simulink model "tremolo"  (R2025b)
settings: Solver=FixedStepDiscrete  StartTime=0.0  StopTime=inf  FixedStep=128/48000  RelTol=1e-3
model workspace (MATLAB code in the model file):
  | Gain_rt = Simulink.Parameter(1.0);
  | Bypass_rt = Simulink.Parameter(false);
undefined symbols (not defined in the file): Depth_rt
settings Model: Creator=linogarciamorales  LastModifiedBy=linogarciamorales
settings OptimizationCC: EnhancedBackFolding=on  PassReuseOutputArgsAs=Individual arguments  ZeroExternalMemoryAtStartup=off  ZeroInternalMemoryAtStartup=off  OptimizeBlockOrder=speed  DifferentSizesBufferReuse=on  OptimizationCustomize=off  EfficientTunableParamExpr=on
settings DebuggingCC: ParameterTunabilityLossMsg=error
settings SFSimCC: MATLABDynamicMemAlloc=off
settings RTWCC: SystemTargetFile=ert.tlc  GenCodeOnly=on  TemplateMakefile=ert_default_tmf  Description=Embedded Coder
settings CodeAppCC: ForceParamTrailComments=on  IgnoreCustomStorageClasses=off  OperatorAnnotations=on  SimulinkDataObjDesc=on  SFDataObjDesc=on  InsertBlockDesc=on
settings ERTTargetCC: InlinedParameterPlacement=Hierarchical  ERTCustomFileTemplate=example_file_process.tlc  TargetLangStandard=C99 (ISO)  GenerateSampleERTMain=on  SupportNonInlinedSFcns=on

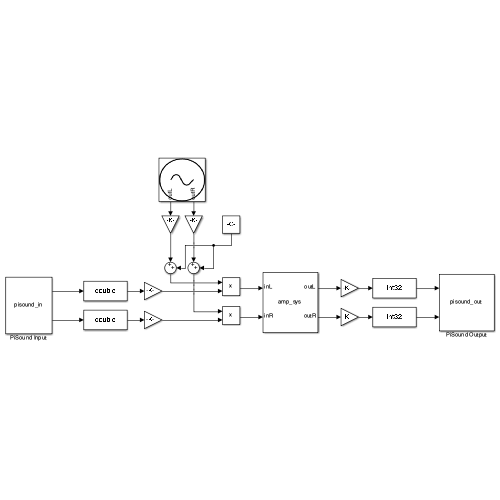
[thumbnail: Simulink's stored preview of the top-level diagram]
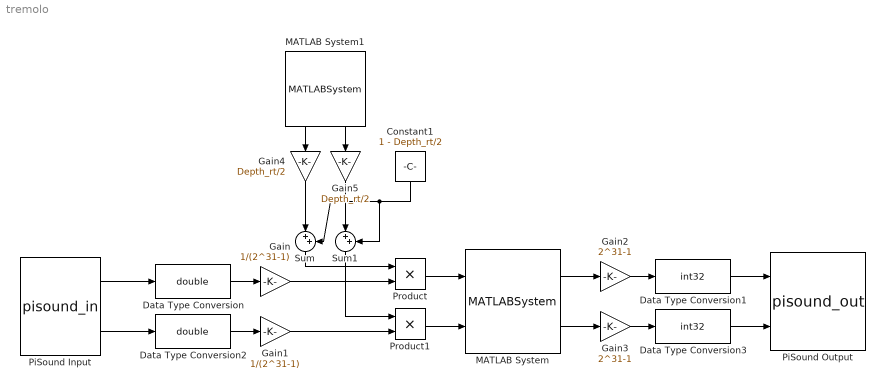
== system tremolo ==
  Constant1 : Constant  Value=1 - Depth_rt/2  OutDataTypeStr=double
  Data Type Conversion : DataTypeConversion  OutDataTypeStr=double  SaturateOnIntegerOverflow=off  RndMeth=Floor
  Data Type Conversion1 : DataTypeConversion  OutDataTypeStr=int32  SaturateOnIntegerOverflow=off  RndMeth=Floor
  Data Type Conversion2 : DataTypeConversion  OutDataTypeStr=double  SaturateOnIntegerOverflow=off  RndMeth=Floor
  Data Type Conversion3 : DataTypeConversion  OutDataTypeStr=int32  SaturateOnIntegerOverflow=off  RndMeth=Floor
  Gain : Gain  Gain=1/(2^31-1)
  Gain1 : Gain  Gain=1/(2^31-1)
  Gain2 : Gain  Gain=2^31-1
  Gain3 : Gain  Gain=2^31-1
  Gain4 : Gain  Gain=Depth_rt/2  ParamDataTypeStr=double
  Gain5 : Gain  Gain=Depth_rt/2  ParamDataTypeStr=double
  MATLAB System : MATLABSystem  System=amp_sys  Fs=48000  Gain=Gain_rt  Bypass=Bypass_rt  SimulateUsing=Code generation
      mask Type: amp_sys
  MATLAB System1 : MATLABSystem  System=osc_sys  N=128  Fs=48000  OutMaxL=4096  InFixL=1024  A=1  F=Rate_rt  iPhase=iPhase_rt  WaveSel=WaveSel_rt  SimulateUsing=Code generation
      mask Type: osc_sys
  PiSound Input : S-Function  FunctionName=pisound_in  Parameters=48000, 128, 0  SFunctionDeploymentMode=off  EnableBusSupport=off
  PiSound Output : S-Function  FunctionName=pisound_out  Parameters=48000, 128, 0  SFunctionDeploymentMode=off  EnableBusSupport=off
  Product : Product  OutDataTypeStr=double
  Product1 : Product  OutDataTypeStr=double
  Sum : Sum  Inputs=|++  OutDataTypeStr=double
  Sum1 : Sum  Inputs=|++  OutDataTypeStr=double
  wires:
  PiSound Input/1 -> Data Type Conversion/1
  Data Type Conversion1/1 -> PiSound Output/1
  Data Type Conversion3/1 -> PiSound Output/2
  Gain2/1 -> Data Type Conversion1/1
  Gain3/1 -> Data Type Conversion3/1
  Data Type Conversion/1 -> Gain/1
  Data Type Conversion2/1 -> Gain1/1
  MATLAB System/1 -> Gain2/1
  MATLAB System/2 -> Gain3/1
  MATLAB System1/1 -> Gain4/1
  Gain/1 -> Product/2
  Sum/1 -> Product/1
  Product/1 -> MATLAB System/1
  Sum1/1 -> Product1/1
  MATLAB System1/2 -> Gain5/1
  Constant1/1 -> Sum1/2, Sum/2
  Gain1/1 -> Product1/2
  Product1/1 -> MATLAB System/2
  Gain4/1 -> Sum/1
  Gain5/1 -> Sum1/1
  PiSound Input/2 -> Data Type Conversion2/1
